simulink model "sampleModel90"  (R2021b)
settings: Solver=VariableStepAuto  StartTime=0.0  StopTime=10.0  RelTol=1e-3
undefined symbols (not defined in the file or in its folder): DiscIntNeverNeededParam, Newton, Raphson
libraries: simulink x16, slpidlib x1
settings Model: Creator=user  LastModifiedBy=user

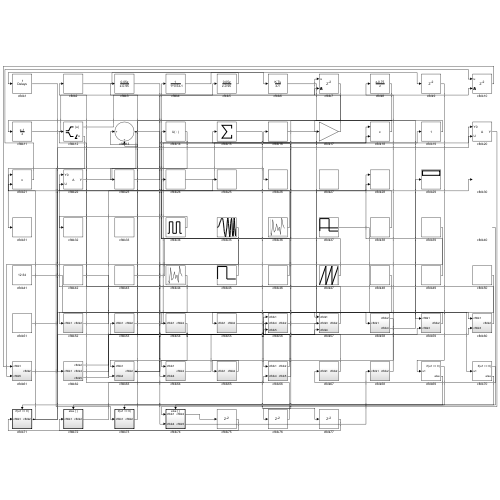
[thumbnail: Simulink's stored preview of the top-level diagram]
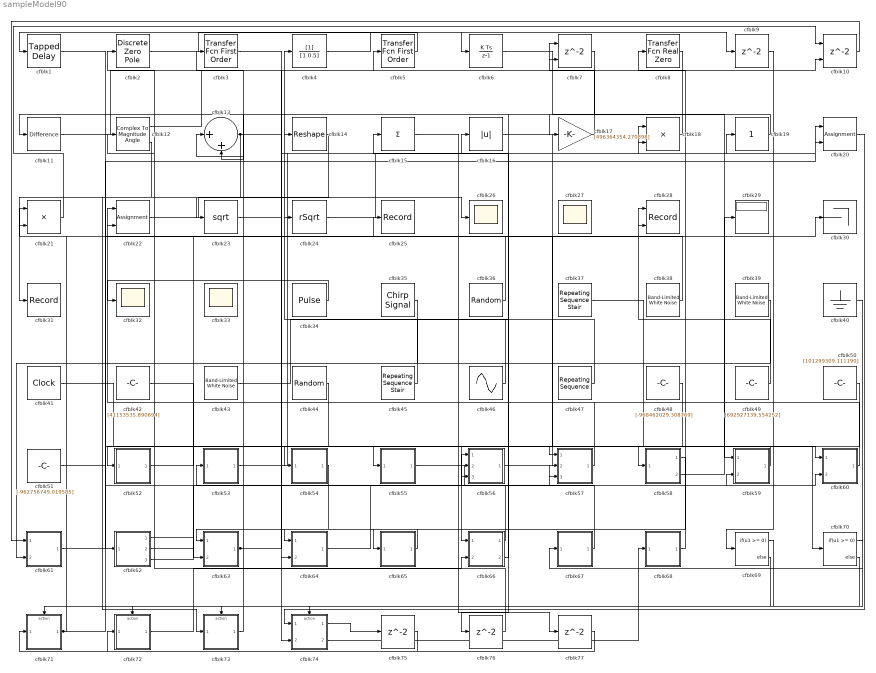
== system sampleModel90 ==
  cfblk1 : simulink/Discrete/Tapped Delay  vinit=0.0  samptime=-1  NumDelays=1  DelayOrder=Oldest  includeCurrent=off
  cfblk10 : Delay  ShowEnablePort=on  SampleTime=1
      settings: InputPortMap=u0,e6
  cfblk11 : simulink/Discrete/Difference  ICPrevInput=0.0  OutMin=[]  OutMax=[]  OutDataTypeStr=Inherit: Inherit via back propagation  OutDataType=fixdt(1, 16)  OutScaling=2^-10  DoSatur=off
  cfblk12 : ComplexToMagnitudeAngle
  cfblk13 : Sum  Inputs=|++
  cfblk14 : Reshape
  cfblk15 : Sum  Inputs=+
  cfblk16 : Abs
  cfblk17 : Gain  Gain=[496364354.270898]
  cfblk18 : Product  Inputs=**
  cfblk19 : simulink/Math Operations/Slider Gain  gain=1  low=0  high=2
  cfblk2 : DiscreteZeroPole  Poles=[0 0.5]  Gain=1
  cfblk20 : Assignment  DiagnosticForDimensions=Warning  IndexOptions=Index vector (dialog)  Indices=1  OutputSizes=1
  cfblk21 : Product  Inputs=**
  cfblk22 : Assignment  DiagnosticForDimensions=Warning  IndexOptions=Index vector (dialog)  Indices=1  OutputSizes=1
  cfblk23 : Sqrt  SaturateOnIntegerOverflow=on
  cfblk24 : Sqrt  Operator=rSqrt  AlgorithmType=Newton-Raphson  SaturateOnIntegerOverflow=on
  cfblk25 : Record  FileSettingsInternal="{\"entries\":[{\"content\":{\"excelSettings\":{\"content\":{},\"type\":\"Streamout.ExcelSettings\"}},\"type\":\"Streamout.FileSettingStorage\",\"uuid\":\"79eebd7f-5a0e-4956-87aa-87d9eb64b5c0\"}],\"packageUris\":[\"http://schema.mathworks.com/mf0/streamout_blocks/R2020a\"],\"version\":\"1.0\"}"  SignalsInternal="{\"entries\":[{\"content\":{\"signals\":[{\"content\":{\"blockPath\":[\"sampleModel90/cfblk25\"],\"channel\":[],\"dimensions\":[1],\"domain\":\"sampleModel90/cfblk25\",\"lineColor\":\"#fe330a\",\"plots\":[1],\"port\":1,\"sid\":[\"\"],\"signalID\":3287,\"signalName\":\"cfblk61\"},\"type\":\"RecordBlkView.Signal\",\"uuid\":\"fbdadaca-47a3-48f0-9cdf-4dd8931d9bce\"}]},\"type\":\"RecordBlkView.InputSignals\",\"uuid\":\"1fe35aa2-7360-4b9c-acdd-d4668150d924\"}],\"packageUris\":[\"http://schema.mathworks.com/mf0/streamout_blocks/R2020a\"],\"version\":\"1.0\"}"  VisualizationBindings="{\"sparklinesplugin\":{\"info\":[{\"bindingParametersList\":[],\"subplotID\":1}]}}"
  cfblk{26..27,32..33} (4 alike) : Scope
      cfblk27 settings: Floating=on
      cfblk33 settings: Floating=on
  cfblk28 : Record  FileSettingsInternal="{\"entries\":[{\"content\":{\"excelSettings\":{\"content\":{},\"type\":\"Streamout.ExcelSettings\"}},\"type\":\"Streamout.FileSettingStorage\",\"uuid\":\"3c84096b-4c15-46d9-a364-f7fda8844328\"}],\"packageUris\":[\"http://schema.mathworks.com/mf0/streamout_blocks/R2020a\"],\"version\":\"1.0\"}"  Layout=[1 1]  SignalsInternal="{\"entries\":[{\"content\":{\"signals\":[{\"content\":{\"blockPath\":[\"sampleModel90/cfblk28\"],\"channel\":[],\"dimensions\":[1],\"domain\":\"sampleModel90/cfblk28\",\"lineColor\":\"#a2142f\",\"plots\":[1],\"port\":1,\"sid\":[\"\"],\"signalID\":3275,\"signalName\":\"cfblk49\"},\"type\":\"RecordBlkView.Signal\",\"uuid\":\"79e036be-4357-4aa0-a290-0a1d569b704f\"},{\"content\":{\"blockPath\":[\"sampleModel90/cfblk28\"],\"channel\":[],\"dimensions\":[1],\"domain\":\"sampleModel90/cfblk28\",\"lineColor\":\"#139fff\",\"plots\":[1],\"port\":2,\"sid\":[\"\"],\"signalID\":3279,\"signalName\":\"cfblk56\"},\"type\":\"RecordBlkView.Signal\",\"uuid\":\"860dffd9-0885-4cff-8dac-714cb6b6142e\"}]},\"type\":\"RecordBlkView.InputSignals\",\"uuid\":\"4815c27b-42a6-4777-83d8-74dd2e280b03\"}],\"packageUris\":[\"http://schema.mathworks.com/mf0/streamout_blocks/R2020a\"],\"version\":\"1.0\"}"  VisualizationBindings="{\"xyplotplugin\":{\"info\":[{\"series\":[{\"bindingParametersList\":[{\"parameter\":\"X-Axis\",\"signalID\":3275,\"signalName\":\"cfblk49\"},{\"parameter\":\"Y-Axis\",\"signalID\":3279,\"signalName\":\"cfblk56\"}],\"seriesID\":34287}],\"subplotID\":1}]}}"  CompatibilityTag=XY
  cfblk29 : Display
  cfblk3 : simulink/Discrete/Transfer Fcn First Order  PoleZ=0.95  ICPrevOutput=0.0  DoSatur=off
  cfblk30 : Terminator
  cfblk31 : Record  FileSettingsInternal="{\"entries\":[{\"content\":{\"excelSettings\":{\"content\":{},\"type\":\"Streamout.ExcelSettings\"}},\"type\":\"Streamout.FileSettingStorage\",\"uuid\":\"9a243126-d6e5-4f53-a83e-323debaafc22\"}],\"packageUris\":[\"http://schema.mathworks.com/mf0/streamout_blocks/R2020a\"],\"version\":\"1.0\"}"  SignalsInternal="{\"entries\":[{\"content\":{\"signals\":[{\"content\":{\"blockPath\":[\"sampleModel90/cfblk31\"],\"channel\":[],\"dimensions\":[1],\"domain\":\"sampleModel90/cfblk31\",\"lineColor\":\"#ff13a6\",\"plots\":[1],\"port\":1,\"sid\":[\"\"],\"signalID\":3283,\"signalName\":\"cfblk13\"},\"type\":\"RecordBlkView.Signal\",\"uuid\":\"c5c4f33c-8707-4618-acaf-1faf330b5491\"}]},\"type\":\"RecordBlkView.InputSignals\",\"uuid\":\"20e3fa54-74c4-4454-b977-684663635461\"}],\"packageUris\":[\"http://schema.mathworks.com/mf0/streamout_blocks/R2020a\"],\"version\":\"1.0\"}"  VisualizationBindings="{\"sparklinesplugin\":{\"info\":[{\"bindingParametersList\":[],\"subplotID\":1}]}}"
  cfblk34 : DiscretePulseGenerator  PulseType=Time based  Amplitude=[-241891757.813479]  Period=[20887671.221871]  PulseWidth=5  PhaseDelay=[2.000000]
  cfblk35 : simulink/Sources/Chirp Signal  f1=[377720666.786466]  T=[326028286.885644]  f2=[-547657205.461768]
  cfblk36 : UniformRandomNumber  Minimum=[-6512285942.847620]  Maximum=[7415139695.582449]  Seed=[10176438.000000]  SampleTime=0.1
  cfblk37 : simulink/Sources/Repeating Sequence Stair  OutValues=[630654758.267392, -221740681.248368]  tsamp=-1  OutMin=[]  OutMax=[]  OutDataTypeStr=double  OutputDataTypeScalingMode=double  OutDataType=fixdt(0,8)  ConRadixGroup=Best Precision: Vector-wise  OutScaling=2^-12
  cfblk38 : simulink/Sources/Band-Limited White Noise  Cov=[3036740754.151934]  Ts=0.1  seed=[8532304677.000000]
  cfblk39 : simulink/Sources/Band-Limited White Noise  Cov=[5708328815.445514]  Ts=0.1  seed=[3505588364.000000]
  cfblk4 : DiscreteFilter  SampleTime=1
  cfblk40 : Ground
  cfblk41 : DigitalClock
  cfblk42 : Constant  Value=[41153535.890694]  SampleTime=1
  cfblk43 : simulink/Sources/Band-Limited White Noise  Cov=[4916625372.734976]  Ts=0.1  seed=[4440977221.000000]
  cfblk44 : UniformRandomNumber  Minimum=[-2085923227.619167]  Maximum=[5468491302.495448]  Seed=[41456488.000000]  SampleTime=0.1
  cfblk45 : simulink/Sources/Repeating Sequence Stair  OutValues=[-540322469.991013, -572384752.950177]  tsamp=-1  OutMin=[]  OutMax=[]  OutDataTypeStr=double  OutputDataTypeScalingMode=double  OutDataType=fixdt(0,8)  ConRadixGroup=Best Precision: Vector-wise  OutScaling=2^-12
  cfblk46 : Sin  Amplitude=[612080064.398325]  Bias=[884281689.453966]  SampleTime=0
  cfblk47 : simulink/Sources/Repeating Sequence  rep_seq_t=[0 2]  rep_seq_y=[-499926153.329129, 681989679.263091]
  cfblk48 : Constant  Value=[-968462029.308769]  SampleTime=1
  cfblk49 : Constant  Value=[692927139.554252]  SampleTime=1
  cfblk5 : simulink/Discrete/Transfer Fcn First Order  PoleZ=0.95  ICPrevOutput=0.0  DoSatur=off
  cfblk50 : Constant  Value=[101299309.111190]  SampleTime=1
  cfblk51 : Constant  Value=[-962756749.019585]  SampleTime=1
  cfblk52 : Subsystem
  cfblk53 : Subsystem
  cfblk54 : Subsystem
  cfblk55 : Subsystem
  cfblk56 : Subsystem
  cfblk57 : Subsystem
  cfblk58 : Subsystem
  cfblk59 : Subsystem
  cfblk6 : DiscreteIntegrator  ICPrevOutput=DiscIntNeverNeededParam  ICPrevScaledInput=DiscIntNeverNeededParam
  cfblk60 : Subsystem
  cfblk61 : Subsystem
  cfblk62 : Subsystem
  cfblk63 : Subsystem
  cfblk64 : Subsystem
  cfblk65 : Subsystem
  cfblk66 : Subsystem
  cfblk67 : Subsystem
  cfblk68 : Subsystem
  cfblk69 : If  IfExpression=u1 >= 0  SampleTime=1
  cfblk7 : Delay  ShowEnablePort=on  SampleTime=1
      settings: InputPortMap=u0,e6
  cfblk70 : If  IfExpression=u1 >= 0  SampleTime=1
  cfblk71 : Subsystem  TreatAsAtomicUnit=on
  cfblk72 : Subsystem  TreatAsAtomicUnit=on
  cfblk73 : Subsystem  TreatAsAtomicUnit=on
  cfblk74 : Subsystem  TreatAsAtomicUnit=on
  cfblk{9,75..77} (4 alike) : Delay  SampleTime=1
  cfblk8 : simulink/Discrete/Transfer Fcn Real Zero  ZeroZ=0.75  ICPrevInput=0.0  DoSatur=off
      settings: SourceProductBaseCode=SL
  wires:
  cfblk36/1 -> cfblk22/1
  cfblk2/1 -> cfblk9/1
  cfblk12/1 -> cfblk5/1
  cfblk12/2 -> cfblk73/1(cfblk1)
  cfblk16/1 -> cfblk60/1(cfblk1)
  cfblk43/1 -> cfblk16/1
  cfblk5/1 -> cfblk1/1
  cfblk66/1(cfblk2) -> cfblk53/1(cfblk1)
  cfblk73/1(cfblk2) -> cfblk13/1
  cfblk52/1(cfblk2) -> cfblk30/1
  cfblk7/1 -> cfblk13/2
  cfblk22/1 -> cfblk26/1
  cfblk50/1 -> cfblk52/1(cfblk1)
  cfblk24/1 -> cfblk18/1
  cfblk55/1(cfblk2) -> cfblk60/2(cfblk3)
  cfblk60/1(cfblk2) -> cfblk22/2
  cfblk18/1 -> cfblk17/1
  cfblk65/1(cfblk2) -> cfblk64/1(cfblk1)
  cfblk63/1(cfblk2) -> cfblk19/1, cfblk57/2(cfblk3)
  cfblk34/1 -> cfblk32/1
  cfblk21/1 -> cfblk10/1
  cfblk6/1 -> cfblk59/1(cfblk1)
  cfblk48/1 -> cfblk66/1(cfblk1)
  cfblk54/1(cfblk2) -> cfblk63/1(cfblk1)
  cfblk10/1 -> cfblk61/1(cfblk1)
  cfblk58/1(cfblk2) -> cfblk65/1(cfblk1)
  cfblk9/1 -> cfblk69/1
  cfblk39/1 -> cfblk61/2(cfblk5)
  cfblk49/1 -> cfblk28/1
  cfblk11/1 -> cfblk7/1
  cfblk13/1 -> cfblk31/1, cfblk20/2
  cfblk68/1(cfblk2) -> cfblk8/1
  cfblk66/2(cfblk5) -> cfblk15/1
  cfblk46/1 -> cfblk4/1
  cfblk1/1 -> cfblk62/1(cfblk1)
  cfblk42/1 -> cfblk63/2(cfblk4)
  cfblk57/1(cfblk2) -> cfblk12/1
  cfblk37/1 -> cfblk70/1
  cfblk40/1 -> cfblk67/1(cfblk1)
  cfblk56/1(cfblk2) -> cfblk28/2
  cfblk14/1 -> cfblk23/1
  cfblk62/1(cfblk2) -> cfblk56/1(cfblk1)
  cfblk58/2(cfblk4) -> cfblk29/1
  cfblk53/1(cfblk2) -> cfblk18/2
  cfblk72/1(cfblk2) -> cfblk66/2(cfblk4)
  cfblk47/1 -> cfblk14/1
  cfblk45/1 -> cfblk24/1
  cfblk51/1 -> cfblk58/1(cfblk1)
  cfblk71/1(cfblk2) -> cfblk21/1, cfblk20/1, cfblk57/3(cfblk4)
  cfblk17/1 -> cfblk7/2
  cfblk64/1(cfblk2) -> cfblk56/2(cfblk4)
  cfblk38/1 -> cfblk21/2
  cfblk19/1 -> cfblk11/1
  cfblk62/2(cfblk4) -> cfblk56/3(cfblk5)
  cfblk44/1 -> cfblk54/1(cfblk1)
  cfblk62/3(cfblk5) -> cfblk59/2(cfblk3)
  cfblk59/1(cfblk2) -> cfblk55/1(cfblk1)
  cfblk4/1 -> cfblk6/1
  cfblk61/1(cfblk2) -> cfblk25/1
  cfblk20/1 -> cfblk74/1(cfblk1)
  cfblk41/1 -> cfblk64/2(cfblk4)
  cfblk35/1 -> cfblk74/2(cfblk4)
  cfblk74/2(cfblk5) -> cfblk68/1(cfblk1)
  cfblk23/1 -> cfblk10/2
  cfblk67/1(cfblk2) -> cfblk3/1
  cfblk3/1 -> cfblk57/1(cfblk1)
  cfblk69/1 -> cfblk71/Action
  cfblk69/2 -> cfblk72/Action
  cfblk70/1 -> cfblk73/Action
  cfblk70/2 -> cfblk74/Action
  cfblk74/1(cfblk2) -> cfblk75/1
  cfblk75/1 -> cfblk71/1(cfblk1)
  cfblk8/1 -> cfblk76/1
  cfblk76/1 -> cfblk2/1
  cfblk15/1 -> cfblk77/1
  cfblk77/1 -> cfblk72/1(cfblk1)

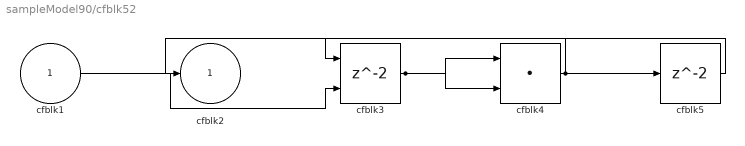
== system sampleModel90/cfblk52 ==
  cfblk1 : Inport
  cfblk3 : Delay  ShowEnablePort=on  SampleTime=1
      settings: InputPortMap=u0,e6
  cfblk4 : DotProduct  InputSameDT=on  OutDataTypeStr=Inherit: Inherit via internal rule
  cfblk5 : Delay  SampleTime=1
  cfblk2 : Outport
  wires:
  cfblk4/1 -> cfblk2/1, cfblk5/1
  cfblk1/1 -> cfblk3/2
  cfblk3/1 -> cfblk4/1, cfblk4/2
  cfblk5/1 -> cfblk3/1

== system sampleModel90/cfblk53 ==
  cfblk1 : Inport
  cfblk3 : Product  Inputs=**
  cfblk2 : Outport
  wires:
  cfblk3/1 -> cfblk2/1
  cfblk1/1 -> cfblk3/1, cfblk3/2

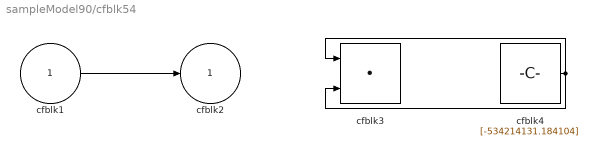
== system sampleModel90/cfblk54 ==
  cfblk1 : Inport
  cfblk3 : DotProduct  InputSameDT=on  OutDataTypeStr=Inherit: Inherit via internal rule
  cfblk4 : Constant  Value=[-534214131.184104]  SampleTime=1
  cfblk2 : Outport
  wires:
  cfblk4/1 -> cfblk3/1, cfblk3/2
  cfblk1/1 -> cfblk2/1

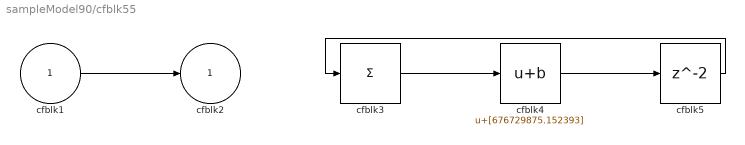
== system sampleModel90/cfblk55 ==
  cfblk1 : Inport
  cfblk3 : Sum  Inputs=+
  cfblk4 : Bias  Bias=[676729875.152393]
  cfblk5 : Delay  SampleTime=1
  cfblk2 : Outport
  wires:
  cfblk1/1 -> cfblk2/1
  cfblk3/1 -> cfblk4/1
  cfblk4/1 -> cfblk5/1
  cfblk5/1 -> cfblk3/1

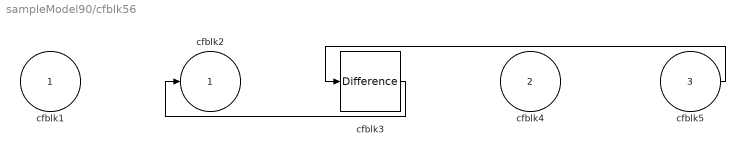
== system sampleModel90/cfblk56 ==
  cfblk1 : Inport
  cfblk4 : Inport  Port=2
  cfblk5 : Inport  Port=3
  cfblk3 : simulink/Discrete/Difference  ICPrevInput=0.0  OutMin=[]  OutMax=[]  OutDataTypeStr=Inherit: Inherit via back propagation  OutDataType=fixdt(1, 16)  OutScaling=2^-10  DoSatur=off
  cfblk2 : Outport
  wires:
  cfblk5/1 -> cfblk3/1
  cfblk3/1 -> cfblk2/1

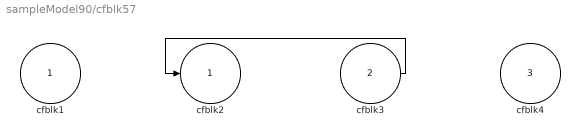
== system sampleModel90/cfblk57 ==
  cfblk1 : Inport
  cfblk3 : Inport  Port=2
  cfblk4 : Inport  Port=3
  cfblk2 : Outport
  wires:
  cfblk3/1 -> cfblk2/1

== system sampleModel90/cfblk58 ==
  cfblk1 : Inport
  cfblk3 : Constant  Value=[541954016.146474]  SampleTime=1
  cfblk2 : Outport
  cfblk4 : Outport  Port=2
  wires:
  cfblk3/1 -> cfblk2/1
  cfblk1/1 -> cfblk4/1

== system sampleModel90/cfblk59 ==
  cfblk1 : Inport
  cfblk3 : Inport  Port=2
  cfblk2 : Outport
  wires:
  cfblk1/1 -> cfblk2/1

== system sampleModel90/cfblk60 ==
  cfblk1 : Inport
  cfblk3 : Inport  Port=2
  cfblk2 : Outport
  wires:
  cfblk1/1 -> cfblk2/1

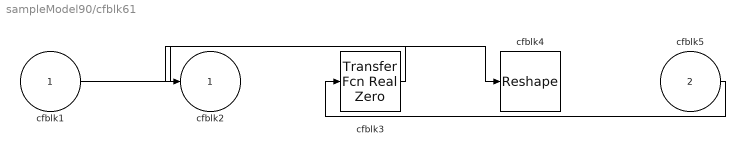
== system sampleModel90/cfblk61 ==
  cfblk1 : Inport
  cfblk5 : Inport  Port=2
  cfblk3 : simulink/Discrete/Transfer Fcn Real Zero  ZeroZ=0.75  ICPrevInput=0.0  DoSatur=off
      settings: SourceProductBaseCode=SL
  cfblk4 : Reshape
  cfblk2 : Outport
  wires:
  cfblk1/1 -> cfblk4/1
  cfblk5/1 -> cfblk3/1
  cfblk3/1 -> cfblk2/1

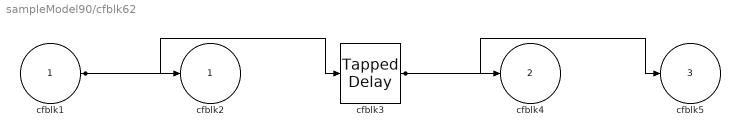
== system sampleModel90/cfblk62 ==
  cfblk1 : Inport
  cfblk3 : simulink/Discrete/Tapped Delay  vinit=0.0  samptime=-1  NumDelays=1  DelayOrder=Oldest  includeCurrent=off
  cfblk2 : Outport
  cfblk4 : Outport  Port=2
  cfblk5 : Outport  Port=3
  wires:
  cfblk1/1 -> cfblk2/1, cfblk3/1
  cfblk3/1 -> cfblk4/1, cfblk5/1

== system sampleModel90/cfblk63 ==
  cfblk1 : Inport
  cfblk4 : Inport  Port=2
  cfblk3 : DiscreteTransferFcn  SampleTime=1
  cfblk2 : Outport
  wires:
  cfblk1/1 -> cfblk3/1
  cfblk4/1 -> cfblk2/1

== system sampleModel90/cfblk64 ==
  cfblk1 : Inport
  cfblk4 : Inport  Port=2
  cfblk3 : ComplexToMagnitudeAngle
  cfblk2 : Outport
  wires:
  cfblk1/1 -> cfblk3/1
  cfblk4/1 -> cfblk2/1

== system sampleModel90/cfblk65 ==
  cfblk1 : Inport
  cfblk3 : DiscreteTransferFcn  SampleTime=1
  cfblk2 : Outport
  wires:
  cfblk1/1 -> cfblk3/1
  cfblk3/1 -> cfblk2/1

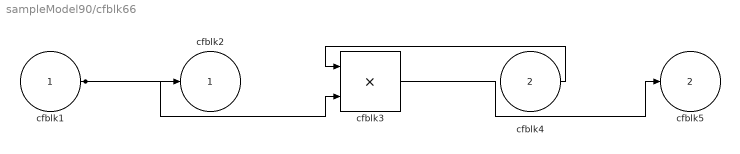
== system sampleModel90/cfblk66 ==
  cfblk1 : Inport
  cfblk4 : Inport  Port=2
  cfblk3 : Product  Inputs=**
  cfblk2 : Outport
  cfblk5 : Outport  Port=2
  wires:
  cfblk4/1 -> cfblk3/1
  cfblk1/1 -> cfblk2/1, cfblk3/2
  cfblk3/1 -> cfblk5/1

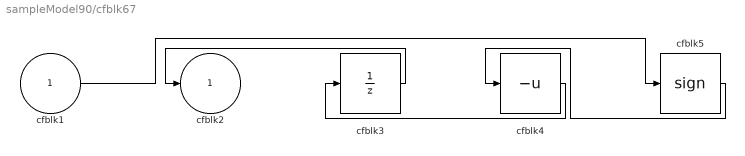
== system sampleModel90/cfblk67 ==
  cfblk1 : Inport
  cfblk3 : UnitDelay  HasFrameUpgradeWarning=on
  cfblk4 : UnaryMinus
  cfblk5 : Signum
  cfblk2 : Outport
  wires:
  cfblk3/1 -> cfblk2/1
  cfblk4/1 -> cfblk3/1
  cfblk1/1 -> cfblk5/1
  cfblk5/1 -> cfblk4/1

== system sampleModel90/cfblk68 ==
  cfblk1 : Inport
  cfblk3 : slpidlib/PID Controller (2DOF)  Controller=PID  Form=Parallel  TimeDomain=Discrete-time  UseExternalTs=off  SampleTime=1  IntegratorMethod=Forward Euler  FilterMethod=Forward Euler  ControllerParametersSource=internal  P=1  I=1  D=0  UseFilter=on  N=100  b=1  c=1  TunerSelectOption=Transfer Function Based (PID Tuner App)  InitialConditionSource=internal  InitialConditionForIntegrator=0  InitialConditionForFilter=0  DifferentiatorICPrevScaledInput=0  ExternalReset=none  TrackingMode=off  Kt=1  LimitOutput=off  SatLimitsSource=internal  UpperSaturationLimit=inf  LowerSaturationLimit=-inf  LinearizeAsGain=off  AntiWindupMode=none  Kb=1  POutMin=[]  POutMax=[]  IOutMin=[]  IOutMax=[]  DOutMin=[]  DOutMax=[]  NOutMin=[]  NOutMax=[]  bOutMin=[]  bOutMax=[]  cOutMin=[]  cOutMax=[]  SumOutMin=[]  SumOutMax=[]  SaturationOutMin=[]  SaturationOutMax=[]  PParamMin=[]  PParamMax=[]  IParamMin=[]  IParamMax=[]  DParamMin=[]  DParamMax=[]  NParamMin=[]  NParamMax=[]  bParamMin=[]  bParamMax=[]  cParamMin=[]  cParamMax=[]  KbParamMin=[]  KbParamMax=[]  KtParamMin=[]  KtParamMax=[]  KbOutMin=[]  KbOutMax=[]  KtOutMin=[]  KtOutMax=[]  IntegratorOutMin=[]  IntegratorOutMax=[]  FilterOutMin=[]  FilterOutMax=[]  SumI1OutMin=[]  SumI1OutMax=[]  SumI2OutMin=[]  SumI2OutMax=[]  SumI3OutMin=[]  SumI3OutMax=[]  SumI4OutMin=[]  SumI4OutMax=[]  SumDOutMin=[]  SumDOutMax=[]  Sum1OutMin=[]  Sum1OutMax=[]  Sum2OutMin=[]  Sum2OutMax=[]  Sum3OutMin=[]  Sum3OutMax=[]  DifferentiatorOutMin=[]  DifferentiatorOutMax=[]  FilterDiffOutCoefMin=[]  FilterDiffOutCoefMax=[]  ReciprocalOutMin=[]  ReciprocalOutMax=[]  SumDenOutMin=[]  SumDenOutMax=[]  SumNumOutMin=[]  SumNumOutMax=[]  DivideOutMin=[]  DivideOutMax=[]  UdiffTsProdOutMin=[]  UdiffTsProdOutMax=[]  NTsProdOutMin=[]  NTsProdOutMax=[]  UintegralTsProdOutMin=[]  UintegralTsProdOutMax=[]  UngainTsProdOutMin=[]  UngainTsProdOutMax=[]  IntegratorContinuousStateAttributes=''  IntegratorStateMustResolveToSignalObject=off  IntegratorRTWStateStorageClass=Auto  FilterContinuousStateAttributes=''  FilterStateMustResolveToSignalObject=off  FilterRTWStateStorageClass=Auto  ParallelPVariant=InternalParameters  IdealPVariant=Disabled  IVariant=InternalParameters  DVariant=InternalParameters  bVariant=InternalParameters  cVariant=InternalParameters  IntegratorVariant=Discrete  SatVariant=Disabled  AWVariant=Passthrough  PCopyVariant=Disabled  TRVariant=Disabled  FdbkBlocksVariant=Forward  IdealPFdbkVariant=Disabled  SatFdbkVariant=Disabled  DerivativeFilterVariant=ForwardEulerFilter  NVariant=InternalParameters  NCopyVariant=Disabled  FilterICVariant=InternalICsFilter  IntegratorICVariant=InternalICs  ExternalResetVariant=Disabled  TRSumVariant=Passthrough  SumFdbkVariant=Disabled  SumVariant=Sum_PID  TsampFilterVariant=InternalTs  TsampNgainVariant=Passthrough  TsampIntegralVariant=Passthrough  ExternalSaturationOutDataTypeStr=Inherit: Same as second input
      settings: SourceProductBaseCode=SL
  cfblk2 : Outport
  wires:
  cfblk1/1 -> cfblk3/1, cfblk3/2
  cfblk3/1 -> cfblk2/1

== system sampleModel90/cfblk71 ==
  cfblk1 : Inport
  Action Port : ActionPort  ActionPortLabel=if(u1 >= 0)
  cfblk3 : DiscreteZeroPole  Poles=[0 0.5]  Gain=1  SampleTime=-1
  cfblk2 : Outport
  wires:
  cfblk1/1 -> cfblk3/1
  cfblk3/1 -> cfblk2/1

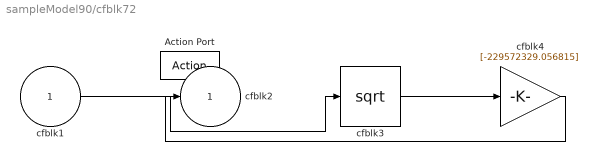
== system sampleModel90/cfblk72 ==
  cfblk1 : Inport
  Action Port : ActionPort  ActionPortLabel=else
  cfblk3 : Sqrt  SaturateOnIntegerOverflow=on
  cfblk4 : Gain  Gain=[-229572329.056815]
  cfblk2 : Outport
  wires:
  cfblk3/1 -> cfblk4/1
  cfblk1/1 -> cfblk3/1
  cfblk4/1 -> cfblk2/1

== system sampleModel90/cfblk73 ==
  cfblk1 : Inport
  Action Port : ActionPort  ActionPortLabel=if(u1 >= 0)
  cfblk3 : Sum  Inputs=-+
  cfblk2 : Outport
  wires:
  cfblk1/1 -> cfblk3/1, cfblk3/2
  cfblk3/1 -> cfblk2/1

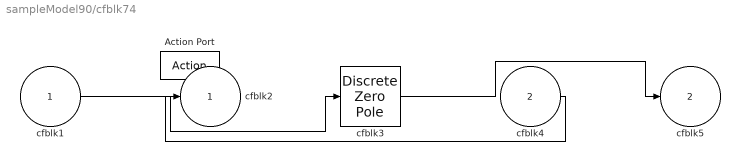
== system sampleModel90/cfblk74 ==
  cfblk1 : Inport
  cfblk4 : Inport  Port=2
  Action Port : ActionPort  ActionPortLabel=else
  cfblk3 : DiscreteZeroPole  Poles=[0 0.5]  Gain=1  SampleTime=-1
  cfblk2 : Outport
  cfblk5 : Outport  Port=2
  wires:
  cfblk1/1 -> cfblk3/1
  cfblk3/1 -> cfblk5/1
  cfblk4/1 -> cfblk2/1
